simulink model "bus_as_currentsource_charging_discharging_battery_1"  (R2023a)
settings: Solver=VariableStepAuto  StartTime=0.0  StopTime=0.01  RelTol=1e-3
libraries: spsParallelRLCBranchLib x72, spsCurrentMeasurementLib x27, spsVoltageMeasurementLib x27, spspowerguiLib x25, spsControlledVoltageSourceLib x24, spsVariableResistorLib x24, spsSeriesRLCBranchLib x6, spsMosfetLib x2, sdolib x1, spsControlledCurrentSourceLib x1, spsGroundLib x1
(part 4 of 4)

== matlab function bus_as_currentsource_charging_discharging_battery_1/Subsystem11/MATLAB Function ==
  data: u input; y output; time input; SOC output; SOC1 input
function [y,SOC]= fcn(u,time,SOC1)
if time <0.006
    SOC= 60 + 60*u/7920;
else
    SOC=SOC1-SOC1*u/7920;
end
y = 5.56e-5.*SOC.^2+0.001788.*SOC+3.491;

== matlab function bus_as_currentsource_charging_discharging_battery_1/Subsystem11/MATLAB Function1 ==
  data: SOC input; y output
function y = fcn(SOC)
p1=2.229e-9;
p2=-5.378e-7;
p3=4.791e-5;
p4=-0.001908;
p5=0.08808;
y=p1*SOC^4+p2*SOC^3+p3*SOC^2+p4*SOC+p5;

== matlab function bus_as_currentsource_charging_discharging_battery_1/Subsystem11/MATLAB Function2 ==
  data: u input; SOC output; time input; SOC1 input
function SOC= fcn(u,time,SOC1)
if time <0.006
    SOC= 60 + 60*u/7920;
else
    SOC=SOC1-SOC1*u/7920;
end

== matlab function bus_as_currentsource_charging_discharging_battery_1/Subsystem12/MATLAB Function ==
  data: u input; y output; time input; SOC output; SOC1 input
function [y,SOC]= fcn(u,time,SOC1)
if time <0.006
    SOC= 60 + 60*u/7920;
else
    SOC=SOC1-SOC1*u/7920;
end
y = 5.56e-5.*SOC.^2+0.001788.*SOC+3.491;

== matlab function bus_as_currentsource_charging_discharging_battery_1/Subsystem12/MATLAB Function1 ==
  data: SOC input; y output
function y = fcn(SOC)
p1=2.229e-9;
p2=-5.378e-7;
p3=4.791e-5;
p4=-0.001908;
p5=0.08808;
y=p1*SOC^4+p2*SOC^3+p3*SOC^2+p4*SOC+p5;

== matlab function bus_as_currentsource_charging_discharging_battery_1/Subsystem12/MATLAB Function2 ==
  data: u input; SOC output; time input; SOC1 input
function SOC= fcn(u,time,SOC1)
if time <0.006
    SOC= 60 + 60*u/7920;
else
    SOC=SOC1-SOC1*u/7920;
end

== matlab function bus_as_currentsource_charging_discharging_battery_1/Subsystem13/MATLAB Function ==
  data: u input; y output; time input; SOC output; SOC1 input
function [y,SOC]= fcn(u,time,SOC1)
if time <0.006
    SOC= 60 + 60*u/7920;
else
    SOC=SOC1-SOC1*u/7920;
end
y = 5.56e-5.*SOC.^2+0.001788.*SOC+3.491;

== matlab function bus_as_currentsource_charging_discharging_battery_1/Subsystem13/MATLAB Function1 ==
  data: SOC input; y output
function y = fcn(SOC)
p1=2.229e-9;
p2=-5.378e-7;
p3=4.791e-5;
p4=-0.001908;
p5=0.08808;
y=p1*SOC^4+p2*SOC^3+p3*SOC^2+p4*SOC+p5;

== matlab function bus_as_currentsource_charging_discharging_battery_1/Subsystem13/MATLAB Function2 ==
  data: u input; SOC output; time input; SOC1 input
function SOC= fcn(u,time,SOC1)
if time <0.006
    SOC= 60 + 60*u/7920;
else
    SOC=SOC1-SOC1*u/7920;
end

== matlab function bus_as_currentsource_charging_discharging_battery_1/Subsystem14/MATLAB Function ==
  data: u input; y output; time input; SOC output; SOC1 input
function [y,SOC]= fcn(u,time,SOC1)
if time <0.006
    SOC= 60 + 60*u/7920;
else
    SOC=SOC1-SOC1*u/7920;
end
y = 5.56e-5.*SOC.^2+0.001788.*SOC+3.491;

== matlab function bus_as_currentsource_charging_discharging_battery_1/Subsystem14/MATLAB Function1 ==
  data: SOC input; y output
function y = fcn(SOC)
p1=2.229e-9;
p2=-5.378e-7;
p3=4.791e-5;
p4=-0.001908;
p5=0.08808;
y=p1*SOC^4+p2*SOC^3+p3*SOC^2+p4*SOC+p5;

== matlab function bus_as_currentsource_charging_discharging_battery_1/Subsystem2/MATLAB Function ==
  data: u input; y output; time input; SOC output; SOC1 input
function [y,SOC]= fcn(u,time,SOC1)
if time <0.006
    SOC= 60 + 60*u/7920;
else
    SOC=SOC1-SOC1*u/7920;
end
y = 5.56e-5.*SOC.^2+0.001788.*SOC+3.491;

== matlab function bus_as_currentsource_charging_discharging_battery_1/Subsystem14/MATLAB Function2 ==
  data: u input; SOC output; time input; SOC1 input
function SOC= fcn(u,time,SOC1)
if time <0.006
    SOC= 60 + 60*u/7920;
else
    SOC=SOC1-SOC1*u/7920;
end

== matlab function bus_as_currentsource_charging_discharging_battery_1/Subsystem15/MATLAB Function ==
  data: u input; y output; time input; SOC output; SOC1 input
function [y,SOC]= fcn(u,time,SOC1)
if time <0.006
    SOC= 60 + 60*u/7920;
else
    SOC=SOC1-SOC1*u/7920;
end
y = 5.56e-5.*SOC.^2+0.001788.*SOC+3.491;

== matlab function bus_as_currentsource_charging_discharging_battery_1/Subsystem15/MATLAB Function1 ==
  data: SOC input; y output
function y = fcn(SOC)
p1=2.229e-9;
p2=-5.378e-7;
p3=4.791e-5;
p4=-0.001908;
p5=0.08808;
y=p1*SOC^4+p2*SOC^3+p3*SOC^2+p4*SOC+p5;

== matlab function bus_as_currentsource_charging_discharging_battery_1/Subsystem15/MATLAB Function2 ==
  data: u input; SOC output; time input; SOC1 input
function SOC= fcn(u,time,SOC1)
if time <0.006
    SOC= 60 + 60*u/7920;
else
    SOC=SOC1-SOC1*u/7920;
end

== matlab function bus_as_currentsource_charging_discharging_battery_1/Subsystem16/MATLAB Function ==
  data: u input; y output; time input; SOC output; SOC1 input
function [y,SOC]= fcn(u,time,SOC1)
if time <0.006
    SOC= 60 + 60*u/7920;
else
    SOC=SOC1-SOC1*u/7920;
end
y = 5.56e-5.*SOC.^2+0.001788.*SOC+3.491;

== matlab function bus_as_currentsource_charging_discharging_battery_1/Subsystem16/MATLAB Function1 ==
  data: SOC input; y output
function y = fcn(SOC)
p1=2.229e-9;
p2=-5.378e-7;
p3=4.791e-5;
p4=-0.001908;
p5=0.08808;
y=p1*SOC^4+p2*SOC^3+p3*SOC^2+p4*SOC+p5;

== matlab function bus_as_currentsource_charging_discharging_battery_1/Subsystem16/MATLAB Function2 ==
  data: u input; SOC output; time input; SOC1 input
function SOC= fcn(u,time,SOC1)
if time <0.006
    SOC= 60 + 60*u/7920;
else
    SOC=SOC1-SOC1*u/7920;
end

== matlab function bus_as_currentsource_charging_discharging_battery_1/Subsystem17/MATLAB Function ==
  data: u input; y output; time input; SOC output; SOC1 input
function [y,SOC]= fcn(u,time,SOC1)
if time <0.006
    SOC= 60 + 60*u/7920;
else
    SOC=SOC1-SOC1*u/7920;
end
y = 5.56e-5.*SOC.^2+0.001788.*SOC+3.491;

== matlab function bus_as_currentsource_charging_discharging_battery_1/Subsystem17/MATLAB Function1 ==
  data: SOC input; y output
function y = fcn(SOC)
p1=2.229e-9;
p2=-5.378e-7;
p3=4.791e-5;
p4=-0.001908;
p5=0.08808;
y=p1*SOC^4+p2*SOC^3+p3*SOC^2+p4*SOC+p5;

== matlab function bus_as_currentsource_charging_discharging_battery_1/Subsystem17/MATLAB Function2 ==
  data: u input; SOC output; time input; SOC1 input
function SOC= fcn(u,time,SOC1)
if time <0.006
    SOC= 60 + 60*u/7920;
else
    SOC=SOC1-SOC1*u/7920;
end

== matlab function bus_as_currentsource_charging_discharging_battery_1/Subsystem18/MATLAB Function ==
  data: u input; y output; time input; SOC output; SOC1 input
function [y,SOC]= fcn(u,time,SOC1)
if time <0.006
    SOC= 60 + 60*u/7920;
else
    SOC=SOC1-SOC1*u/7920;
end
y = 5.56e-5.*SOC.^2+0.001788.*SOC+3.491;

== matlab function bus_as_currentsource_charging_discharging_battery_1/Subsystem2/MATLAB Function1 ==
  data: SOC input; y output
function y = fcn(SOC)
p1=2.229e-9;
p2=-5.378e-7;
p3=4.791e-5;
p4=-0.001908;
p5=0.08808;
y=p1*SOC^4+p2*SOC^3+p3*SOC^2+p4*SOC+p5;

== matlab function bus_as_currentsource_charging_discharging_battery_1/Subsystem18/MATLAB Function1 ==
  data: SOC input; y output
function y = fcn(SOC)
p1=2.229e-9;
p2=-5.378e-7;
p3=4.791e-5;
p4=-0.001908;
p5=0.08808;
y=p1*SOC^4+p2*SOC^3+p3*SOC^2+p4*SOC+p5;

== matlab function bus_as_currentsource_charging_discharging_battery_1/Subsystem18/MATLAB Function2 ==
  data: u input; SOC output; time input; SOC1 input
function SOC= fcn(u,time,SOC1)
if time <0.006
    SOC= 60 + 60*u/7920;
else
    SOC=SOC1-SOC1*u/7920;
end

== matlab function bus_as_currentsource_charging_discharging_battery_1/Subsystem19/MATLAB Function ==
  data: u input; y output; time input; SOC output; SOC1 input
function [y,SOC]= fcn(u,time,SOC1)
if time <0.006
    SOC= 60 + 60*u/7920;
else
    SOC=SOC1-SOC1*u/7920;
end
y = 5.56e-5.*SOC.^2+0.001788.*SOC+3.491;

== matlab function bus_as_currentsource_charging_discharging_battery_1/Subsystem19/MATLAB Function1 ==
  data: SOC input; y output
function y = fcn(SOC)
p1=2.229e-9;
p2=-5.378e-7;
p3=4.791e-5;
p4=-0.001908;
p5=0.08808;
y=p1*SOC^4+p2*SOC^3+p3*SOC^2+p4*SOC+p5;

== matlab function bus_as_currentsource_charging_discharging_battery_1/Subsystem19/MATLAB Function2 ==
  data: u input; SOC output; time input; SOC1 input
function SOC= fcn(u,time,SOC1)
if time <0.006
    SOC= 60 + 60*u/7920;
else
    SOC=SOC1-SOC1*u/7920;
end

== matlab function bus_as_currentsource_charging_discharging_battery_1/Subsystem20/MATLAB Function ==
  data: u input; y output; time input; SOC output; SOC1 input
function [y,SOC]= fcn(u,time,SOC1)
if time <0.006
    SOC= 60 + 60*u/7920;
else
    SOC=SOC1-SOC1*u/7920;
end
y = 5.56e-5.*SOC.^2+0.001788.*SOC+3.491;

== matlab function bus_as_currentsource_charging_discharging_battery_1/Subsystem20/MATLAB Function1 ==
  data: SOC input; y output
function y = fcn(SOC)
p1=2.229e-9;
p2=-5.378e-7;
p3=4.791e-5;
p4=-0.001908;
p5=0.08808;
y=p1*SOC^4+p2*SOC^3+p3*SOC^2+p4*SOC+p5;

== matlab function bus_as_currentsource_charging_discharging_battery_1/Subsystem20/MATLAB Function2 ==
  data: u input; SOC output; time input; SOC1 input
function SOC= fcn(u,time,SOC1)
if time <0.006
    SOC= 60 + 60*u/7920;
else
    SOC=SOC1-SOC1*u/7920;
end

== matlab function bus_as_currentsource_charging_discharging_battery_1/Subsystem2/MATLAB Function2 ==
  data: u input; SOC output; time input; SOC1 input
function SOC= fcn(u,time,SOC1)
if time <0.006
    SOC= 60 + 60*u/7920;
else
    SOC=SOC1-SOC1*u/7920;
end

== matlab function bus_as_currentsource_charging_discharging_battery_1/Subsystem21/MATLAB Function ==
  data: u input; y output; time input; SOC output; SOC1 input
function [y,SOC]= fcn(u,time,SOC1)
if time <0.006
    SOC= 60 + 60*u/7920;
else
    SOC=SOC1-SOC1*u/7920;
end
y = 5.56e-5.*SOC.^2+0.001788.*SOC+3.491;

== matlab function bus_as_currentsource_charging_discharging_battery_1/Subsystem21/MATLAB Function1 ==
  data: SOC input; y output
function y = fcn(SOC)
p1=2.229e-9;
p2=-5.378e-7;
p3=4.791e-5;
p4=-0.001908;
p5=0.08808;
y=p1*SOC^4+p2*SOC^3+p3*SOC^2+p4*SOC+p5;

== matlab function bus_as_currentsource_charging_discharging_battery_1/Subsystem21/MATLAB Function2 ==
  data: u input; SOC output; time input; SOC1 input
function SOC= fcn(u,time,SOC1)
if time <0.006
    SOC= 60 + 60*u/7920;
else
    SOC=SOC1-SOC1*u/7920;
end

== matlab function bus_as_currentsource_charging_discharging_battery_1/Subsystem22/MATLAB Function ==
  data: u input; y output; time input; SOC output; SOC1 input
function [y,SOC]= fcn(u,time,SOC1)
if time <0.006
    SOC= 60 + 60*u/7920;
else
    SOC=SOC1-SOC1*u/7920;
end
y = 5.56e-5.*SOC.^2+0.001788.*SOC+3.491;

== matlab function bus_as_currentsource_charging_discharging_battery_1/Subsystem22/MATLAB Function1 ==
  data: SOC input; y output
function y = fcn(SOC)
p1=2.229e-9;
p2=-5.378e-7;
p3=4.791e-5;
p4=-0.001908;
p5=0.08808;
y=p1*SOC^4+p2*SOC^3+p3*SOC^2+p4*SOC+p5;

== matlab function bus_as_currentsource_charging_discharging_battery_1/Subsystem22/MATLAB Function2 ==
  data: u input; SOC output; time input; SOC1 input
function SOC= fcn(u,time,SOC1)
if time <0.006
    SOC= 60 + 60*u/7920;
else
    SOC=SOC1-SOC1*u/7920;
end

== matlab function bus_as_currentsource_charging_discharging_battery_1/Subsystem23/MATLAB Function ==
  data: u input; y output; time input; SOC output; SOC1 input
function [y,SOC]= fcn(u,time,SOC1)
if time <0.006
    SOC= 60 + 60*u/7920;
else
    SOC=SOC1-SOC1*u/7920;
end
y = 5.56e-5.*SOC.^2+0.001788.*SOC+3.491;

== matlab function bus_as_currentsource_charging_discharging_battery_1/Subsystem23/MATLAB Function1 ==
  data: SOC input; y output
function y = fcn(SOC)
p1=2.229e-9;
p2=-5.378e-7;
p3=4.791e-5;
p4=-0.001908;
p5=0.08808;
y=p1*SOC^4+p2*SOC^3+p3*SOC^2+p4*SOC+p5;

== matlab function bus_as_currentsource_charging_discharging_battery_1/Subsystem23/MATLAB Function2 ==
  data: u input; SOC output; time input; SOC1 input
function SOC= fcn(u,time,SOC1)
if time <0.006
    SOC= 60 + 60*u/7920;
else
    SOC=SOC1-SOC1*u/7920;
end

== matlab function bus_as_currentsource_charging_discharging_battery_1/MATLAB Function ==
  data: u input; y output
function y = fcn(u)

if u<0.002
    y=200/24*u/0.002;
elseif u<0.004
    y=200/24;
elseif u<0.008
    y=200/24*(3-500*u);
else
    y=-200/24;
end

== matlab function bus_as_currentsource_charging_discharging_battery_1/MATLAB Function1 ==
  data: btv input; duty output; current input
function duty = fcn(btv,current)
if current<0
    duty=1-24/btv;
else
    duty=24/btv;
end

== matlab function bus_as_currentsource_charging_discharging_battery_1/Subsystem3/MATLAB Function ==
  data: u input; y output; time input; SOC output; SOC1 input
function [y,SOC]= fcn(u,time,SOC1)
if time <0.006
    SOC= 60 + 60*u/7920;
else
    SOC=SOC1-SOC1*u/7920;
end
y = 5.56e-5.*SOC.^2+0.001788.*SOC+3.491;

== matlab function bus_as_currentsource_charging_discharging_battery_1/MATLAB Function2 ==
  data: u input; y output; time input
function y = fcn(u,time)
if time>0.006 & time<0.0065
    y=double(0);
else
    y = double(u);
end

== matlab function bus_as_currentsource_charging_discharging_battery_1/MATLAB Function3 ==
  data: u input; y output; time input
function y = fcn(u,time)
if time>0.006 & time<0.0065
    y=double(0);
else
    y = double(u);
end

== matlab function bus_as_currentsource_charging_discharging_battery_1/Subsystem24/MATLAB Function ==
  data: u input; y output; time input; SOC output; SOC1 input
function [y,SOC]= fcn(u,time,SOC1)
if time <0.006
    SOC= 60 + 60*u/7920;
else
    SOC=SOC1-SOC1*u/7920;
end
y = 5.56e-5.*SOC.^2+0.001788.*SOC+3.491;

== matlab function bus_as_currentsource_charging_discharging_battery_1/Subsystem24/MATLAB Function1 ==
  data: SOC input; y output
function y = fcn(SOC)
p1=2.229e-9;
p2=-5.378e-7;
p3=4.791e-5;
p4=-0.001908;
p5=0.08808;
y=p1*SOC^4+p2*SOC^3+p3*SOC^2+p4*SOC+p5;

== matlab function bus_as_currentsource_charging_discharging_battery_1/Subsystem24/MATLAB Function2 ==
  data: u input; SOC output; time input; SOC1 input
function SOC= fcn(u,time,SOC1)
if time <0.006
    SOC= 60 + 60*u/7920;
else
    SOC=SOC1-SOC1*u/7920;
end

== matlab function bus_as_currentsource_charging_discharging_battery_1/Subsystem3/MATLAB Function1 ==
  data: SOC input; y output
function y = fcn(SOC)
p1=2.229e-9;
p2=-5.378e-7;
p3=4.791e-5;
p4=-0.001908;
p5=0.08808;
y=p1*SOC^4+p2*SOC^3+p3*SOC^2+p4*SOC+p5;

== matlab function bus_as_currentsource_charging_discharging_battery_1/Subsystem3/MATLAB Function2 ==
  data: u input; SOC output; time input; SOC1 input
function SOC= fcn(u,time,SOC1)
if time <0.006
    SOC= 60 + 60*u/7920;
else
    SOC=SOC1-SOC1*u/7920;
end

== matlab function bus_as_currentsource_charging_discharging_battery_1/Subsystem4/MATLAB Function ==
  data: u input; y output; time input; SOC output; SOC1 input
function [y,SOC]= fcn(u,time,SOC1)
if time <0.006
    SOC= 60 + 60*u/7920;
else
    SOC=SOC1-SOC1*u/7920;
end
y = 5.56e-5.*SOC.^2+0.001788.*SOC+3.491;

== matlab function bus_as_currentsource_charging_discharging_battery_1/Subsystem4/MATLAB Function1 ==
  data: SOC input; y output
function y = fcn(SOC)
p1=2.229e-9;
p2=-5.378e-7;
p3=4.791e-5;
p4=-0.001908;
p5=0.08808;
y=p1*SOC^4+p2*SOC^3+p3*SOC^2+p4*SOC+p5;
